simulink model "TractiveSystemCooling"  (R2023b)
settings: Solver=FixedStepAuto  StartTime=0.0  StopTime=runtime  FixedStep=.02  RelTol=1e-3
model workspace: external: MATLAB File Data/Settings.m (data not in the file)
undefined symbols (not defined in the file or in its folder): Cell, runtime, TSAC
libraries: fl_lib x5, nesl_utility x5, batteryecm_lib x1, dspstat3 x1
settings Model: Creator=13359

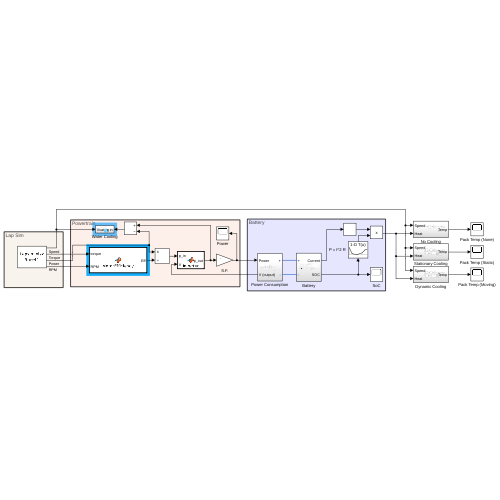
[thumbnail: Simulink's stored preview of the top-level diagram]
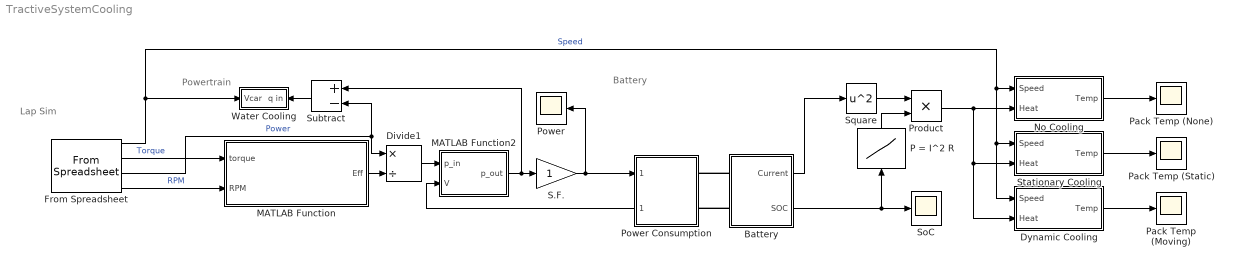
== system TractiveSystemCooling ==
  note: Powertrain
  note: Battery
  note: Lap Sim
  Battery : Subsystem
  Divide1 : Product  Inputs=*/
  Dynamic Cooling : Subsystem
  From Spreadsheet : FromSpreadsheet  FileName=Lapsim.xlsx  Range=E1:E5414, W1:Y5414  TreatFirstColumnAs=Data  SampleTime=0.02
  MATLAB Function : MATLAB Function  TreatAsAtomicUnit=on
  MATLAB Function2 : MATLAB Function  TreatAsAtomicUnit=on
  No Cooling : Subsystem
  P = I^2 R : Lookup_n-D  NumberOfTableDimensions=1  BreakpointsForDimension1=Cell.SOC  Table=zeros(1,length(Cell.SOC)) + (Cell.Resistance*Cell.series/Cell.parallel)  InternalRulePriority=Speed  RndMeth=Simplest
  Pack Temp (Moving) : Scope
  Pack Temp (None) : Scope
  Pack Temp (Static) : Scope
  Power : Scope
  Power Consumption : Subsystem
      settings: PortSchema="{\"entries\":[{\"content\":{\"sides\":[{\"content\":{\"connectorIds\":[\"In1\",\"Out1\"]},\"type\":\"ConnectorPlacement.EquallySpacedRectSide\",\"uuid\":\"bce31be9-9828-45d3-a0ec-acfed125f971\"},{\"content\":{\"connectorIds\":[\"RConn1\",\"RConn2\"],\"side\":\"RIGHT\"},\"type\":\"ConnectorPlacement.EquallySpacedRectSide\",\"uuid\":\"688da906-5253-49d4-8895-2a1ab7d3d08f\"},{\"content\":{\"side\":\"TOP\"},\"type\":\"ConnectorPlacement.EquallySpacedRectSide\",\"uuid\":\"26fec6ea-0e9b-46d7-ab73-190f763a0feb\"}]},\"type\":\"ConnectorPlacement.EquallySpacedConnector\",\"uuid\":\"dca3bc88-c6e8-4b99-b46a-70a0164d4b50\"}],\"packageUris\":[\"http://schema.mathworks.com/mf0/Connector/R2020b\"],\"version\":\"1.0\"}"
  Product : Product
  S.F. : Gain
  SoC : Scope
  Square : Math  Operator=square
  Stationary Cooling : Subsystem
  Subtract : Sum  Inputs=+-
  Water Cooling : Subsystem
      settings: PortSchema="{\"entries\":[{\"content\":{\"sides\":[{\"content\":{\"connectorIds\":[\"In1\"]},\"type\":\"ConnectorPlacement.EquallySpacedRectSide\",\"uuid\":\"7b584cd1-b16c-47c3-a77c-0f72b30f83a9\"},{\"content\":{\"connectorIds\":[\"In2\"],\"side\":\"RIGHT\"},\"type\":\"ConnectorPlacement.EquallySpacedRectSide\",\"uuid\":\"743ce824-323e-45dd-9a42-fd02d44e7a7c\"},{\"content\":{\"side\":\"TOP\"},\"type\":\"ConnectorPlacement.EquallySpacedRectSide\",\"uuid\":\"adabee87-d3a0-4ce2-a1ff-e6a273d4f474\"}]},\"type\":\"ConnectorPlacement.EquallySpacedConnector\",\"uuid\":\"782a8077-db8b-432e-a7e4-fc43f04762f2\"}],\"packageUris\":[\"http://schema.mathworks.com/mf0/Connector/R2020b\"],\"version\":\"1.0\"}"
  wires:
  MATLAB Function/1(Eff) -> Divide1/2
  From Spreadsheet/3 -> Divide1/1, Subtract/2  "Power"
  From Spreadsheet/2 -> MATLAB Function/1(torque)  "Torque"
  Square/1 -> Product/1
  From Spreadsheet/4 -> MATLAB Function/2(RPM)  "RPM"
  Product/1 -> Stationary Cooling/2(Heat), Dynamic Cooling/2(Heat), No Cooling/2(Heat)
  S.F./1 -> Power/1, Power Consumption/1(Power)
  From Spreadsheet/1 -> Dynamic Cooling/1(Speed), Stationary Cooling/1(Speed), No Cooling/1(Speed), Water Cooling/2(Vcar)  "Speed"
  Subtract/1 -> Water Cooling/1(q in)
  Divide1/1 -> MATLAB Function2/1(p_in)
  MATLAB Function2/1(p_out) -> S.F./1, Subtract/1
  Dynamic Cooling/1(Temp) -> Pack Temp (Moving)/1
  Stationary Cooling/1(Temp) -> Pack Temp (Static)/1
  No Cooling/1(Temp) -> Pack Temp (None)/1
  Battery/2(SOC) -> P = I^2 R/1, SoC/1
  Power Consumption/1(V (output)) -> MATLAB Function2/2(V)
  P = I^2 R/1 -> Product/2
  Battery/1(Current) -> Square/1
  connections:
  Battery/LConn2 -- Power Consumption/RConn2
  Battery/LConn1 -- Power Consumption/RConn1

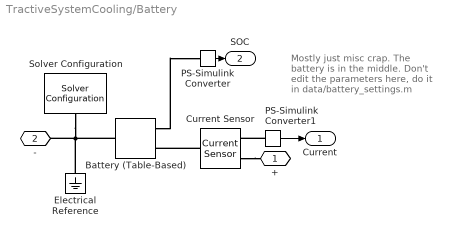
== system TractiveSystemCooling/Battery ==
  note: Mostly just misc crap.
      | The battery is in the
      | middle. Don't edit the
      | parameters here, do it
      | in data/battery_settings.m
  Battery (Table-Based) : batteryecm_lib/Battery (Table-Based)  SOC_vec=Cell.SOC  T_dependence=simscape.enum.tablebattery.temperature_dependence.no  prm_dir=simscape.enum.tablebattery.prm_dir.noCurrentDirectionality  T_vec=[278, 293, 313] K  V0_mat=[3.49, 3.5, 3.51; 3.55, 3.57, 3.56; 3.62, 3.63, 3.64; 3.71, 3.71, 3.72; 3.91, 3.93, 3.94; 4.07, 4.08, 4.08; 4.19, 4.19, 4.19] V  V0_vec=zeros(1,length(Cell.SOC)) + (Cell.V * Cell.series) V  V_range=[0, inf] V  R0_mat=[.0117, .0085, .009; .011, .0085, .009; .0114, .0087, .0092; .0107, .0082, .0088; .0107, .0083, .0091; .0113, .0085, .0089; .0116, .0085, .0089] Ohm  R0_vec=zeros(1,length(Cell.SOC)) + (Cell.Resistance*Cell.series/Cell.parallel) Ohm  R0_dis_mat=[.0117, .0085, .009; .011, .0085, .009; .0114, .0087, .0092; .0107, .0082, .0088; .0107, .0083, .0091; .0113, .0085, .0089; .0116, .0085, .0089] Ohm  R0_dis_vec=[.0085, .0085, .0087, .0082, .0083, .0085, .0085] Ohm  R0_ch_mat=[.0117, .0085, .009; .011, .0085, .009; .0114, .0087, .0092; .0107, .0082, .0088; .0107, .0083, .0091; .0113, .0085, .0089; .0116, .0085, .0089] Ohm  R0_ch_vec=[.0085, .0085, .0087, .0082, .0083, .0085, .0085] Ohm  AH=Cell.Capacity * Cell.parallel A*hr  prm_leak=simscape.enum.tablebattery.prm_leak.disabled  Rleak_vec=[8000, 7000, 6000] Ohm  Rleak=7e3 Ohm  extrapolation_option=simscape.enum.extrapolation.linear  SOC_port=simscape.enum.tablebattery.enable.yes  prm_dyn=simscape.enum.tablebattery.prm_dyn.off  R1_mat=[.0109, .0029, .0013; .0069, .0024, .0012; .0047, .0026, .0013; .0034, .0016, .001; .0033, .0023, .0014; .0033, .0018, .0011; .0028, .0017, .0011] Ohm  R1_vec=[.0029, .0024, .0026, .0016, .0023, .0018, .0017] Ohm  tau1_mat=[20, 36, 39; 31, 45, 39; 109, 105, 61; 36, 29, 26; 59, 77, 67; 40, 33, 29; 25, 39, 33] s  tau1_vec=[36, 45, 105, 29, 77, 33, 39] s  R2_mat=[.0109, .0029, .0013; .0069, .0024, .0012; .0047, .0026, .0013; .0034, .0016, .001; .0033, .0023, .0014; .0033, .0018, .0011; .0028, .0017, .0011] Ohm  R2_vec=[.0029, .0024, .0026, .0016, .0023, .0018, .0017] Ohm  tau2_mat=[20, 36, 39; 31, 45, 39; 109, 105, 61; 36, 29, 26; 59, 77, 67; 40, 33, 29; 25, 39, 33] s  tau2_vec=[36, 45, 105, 29, 77, 33, 39] s  R3_mat=[.0109, .0029, .0013; .0069, .0024, .0012; .0047, .0026, .0013; .0034, .0016, .001; .0033, .0023, .0014; .0033, .0018, .0011; .0028, .0017, .0011] Ohm  R3_vec=[.0029, .0024, .0026, .0016, .0023, .0018, .0017] Ohm  tau3_mat=[20, 36, 39; 31, 45, 39; 109, 105, 61; 36, 29, 26; 59, 77, 67; 40, 33, 29; 25, 39, 33] s  tau3_vec=[36, 45, 105, 29, 77, 33, 39] s  R4_mat=[.0109, .0029, .0013; .0069, .0024, .0012; .0047, .0026, .0013; .0034, .0016, .001; .0033, .0023, .0014; .0033, .0018, .0011; .0028, .0017, .0011] Ohm  R4_vec=[.0029, .0024, .0026, .0016, .0023, .0018, .0017] Ohm  tau4_mat=[20, 36, 39; 31, 45, 39; 109, 105, 61; 36, 29, 26; 59, 77, 67; 40, 33, 29; 25, 39, 33] s  tau4_vec=[36, 45, 105, 29, 77, 33, 39] s  R5_mat=[.0109, .0029, .0013; .0069, .0024, .0012; .0047, .0026, .0013; .0034, .0016, .001; .0033, .0023, .0014; .0033, .0018, .0011; .0028, .0017, .0011] Ohm  R5_vec=[.0029, .0024, .0026, .0016, .0023, .0018, .0017] Ohm  tau5_mat=[20, 36, 39; 31, 45, 39; 109, 105, 61; 36, 29, 26; 59, 77, 67; 40, 33, 29; 25, 39, 33] s  tau5_vec=[36, 45, 105, 29, 77, 33, 39] s  prm_fade=simscape.enum.tablebattery.prm_fade.disabled  N0=100  dV0=0  dR0=0  dAH=0  dRleak=0  dR1=0  dR2=0  dR3=0  dR4=0  dR5=0  N0vec=[0, 100, 200, 300]  Tfadevec=[298.15, 323.15] K  dV0vec=[0, 0, 0, 0]  dR0vec=[0, 0, 0, 0]  dAHvec=[0, 0, 0, 0]  dRleakvec=[0, 0, 0, 0]  dR1vec=[0, 0, 0, 0]  dR2vec=[0, 0, 0, 0]  dR3vec=[0, 0, 0, 0]  dR4vec=[0, 0, 0, 0]  dR5vec=[0, 0, 0, 0]  dV0mat=[0, 0; 0, 0; 0, 0; 0, 0]  dR0mat=[0, 0; 0, 0; 0, 0; 0, 0]  dAHmat=[0, 0; 0, 0; 0, 0; 0, 0]  dRleakmat=[0, 0; 0, 0; 0, 0; 0, 0]  dR1mat=[0, 0; 0, 0; 0, 0; 0, 0]  dR2mat=[0, 0; 0, 0; 0, 0; 0, 0]  dR3mat=[0, 0; 0, 0; 0, 0; 0, 0]  dR4mat=[0, 0; 0, 0; 0, 0; 0, 0]  dR5mat=[0, 0; 0, 0; 0, 0; 0, 0]  prm_age_modeling=simscape.enum.tablebattery.prm_age_modeling.equation  storage_dt_age_vec=[0] d  storage_T_age_vec=[273] K  prm_age_OCV=simscape.enum.tablebattery.prm_age_OCV.OCV  OCV_age=0.9  SOC_age=0.6  prm_age_resistance=simscape.enum.tablebattery.prm_age.disabled  OCV_scaling_age_resistance=2.2134e6  OCV_offset_age_resistance=1.632e6  temp_exp_age_resistance=0.515833569 V  t_exp_age_resistance=0.75  T_age_vec_resistance=[273.15, 298.15, 323.15] K  dt_age_vec_resistance=[0, 90, 180, 270] d  dR0_age_vec=[0, 0, 0]  t_meas_dR0_age=100 d  dR0_age_mat=[0, 0, 0; 0, 0, 0; 0, 0, 0; 0, 0, 0]  prm_age_capacity=simscape.enum.tablebattery.prm_age.disabled  OCV_scaling_age_capacity=1.5097e07  OCV_offset_age_capacity=8.3625e06  temp_exp_age_capacity=0.6011 V  t_exp_age_capacity=0.75  T_age_vec_capacity=[273.15, 298.15, 323.15] K  dt_age_vec_capacity=[0, 90, 180, 270] d  dAH_age_vec=[0, 0, 0]  t_meas_dAH_age=100 d  dAH_age_mat=[0, 0, 0; 0, 0, 0; 0, 0, 0; 0, 0, 0]  thermal_port=simscape.enum.thermaleffects.omit  temperature=298.15 K  thermal_mass=100 J/K  i_specify=off  i_priority=None  i=0 A  i_nominal_specify=off  i_nominal_unit=A  i_nominal_value=1  v_specify=off  v_priority=None  v=0 V  v_nominal_specify=off  v_nominal_unit=V  v_nominal_value=1  stateOfCharge_specify=off  stateOfCharge_priority=High  stateOfCharge=1  stateOfCharge_nominal_specify=off  stateOfCharge_nominal_unit=1  stateOfCharge_nominal_value=1  num_cycles_specify=off  num_cycles_priority=High  num_cycles=0  num_cycles_nominal_specify=off  num_cycles_nominal_unit=1  num_cycles_nominal_value=1  cell_temperature_specify=off  cell_temperature_priority=High  cell_temperature=298.15 K  cell_temperature_nominal_specify=off  cell_temperature_nominal_unit=K  cell_temperature_nominal_value=1
      settings: InternalSimscapePortConfiguration="{\"Bottom\":[],\"Left\":[{\"id\":\"p\",\"label\":\"+\",\"type\":\"foundation.electrical.electrical\"},{\"id\":\"soc\",\"label\":\"SOC\",\"type\":\"output\"}],\"Right\":[{\"id\":\"n\",\"label\":\"-\",\"type\":\"foundation.electrical.electrical\"}],\"Top\":[]}"
      settings: LibrarySourceBlock=|
      | batt_lib/Cells/Battery
      | (Table-Based)
  Current Sensor : fl_lib/Electrical/Electrical Sensors/Current Sensor
  Electrical Reference : fl_lib/Electrical/Electrical Elements/Electrical Reference
  PS-Simulink Converter : nesl_utility/PS-Simulink Converter  PhysicalDomain=network_engine_domain  SubClassName=ps_output  LeftPortType=input  RightPortType=output  PseudoPeriodic=off  Frequencies=[]  VectorFormat=inherit  Unit=inherit  AffineConversion=off
  PS-Simulink Converter1 : nesl_utility/PS-Simulink Converter  PhysicalDomain=network_engine_domain  SubClassName=ps_output  LeftPortType=input  RightPortType=output  PseudoPeriodic=off  Frequencies=[]  VectorFormat=inherit  Unit=inherit  AffineConversion=off
  Solver Configuration : nesl_utility/Solver Configuration  PhysicalDomain=network_engine_domain  SubClassName=solver  LeftPortType=input  RightPortType=generic  Tones=[]  Harmonics=[]  SimulateNoise=off  Profile=off  UseLocalSampling=off  EnableSwitchedLinearOptims=on  FrequencyDomain=off  UseCCode=off  RelTol=0.001  AbsTol=0.001  MinStep=1e-09  ToWorkspace=off  RevertToSquareIcSolve=off  NumHomotopyIterations=100  PhasorMode=off  PhasorModeNumHarmonics=1  ConsistencySolver=NEWTON_XTOL_AFTER_FTOL  IndexReductionMethod=DerivativeReplacement  DoDC=off  ResidualTolerance=1e-09  ConsistencyTolSource=GLOBAL  ConsistencyAbsTol=0.001  ConsistencyRelTol=0.001  ConsistencyTolFactor=0.001  UseLocalSolver=on  LocalSolverChoice=NE_BACKWARD_EULER_ADVANCER  ResolveIndetEquations=on  FunctionEvalNumThread=1  LocalSolverSampleTime=0.02  DoFixedCost=on  MaxNonlinIter=3  MaxModeIter=2  ComputeImpulses=off  ImpulseIterations=2  LinearAlgebra=auto  LinearAlgebraNumThread=0  EquationFormulation=NE_TIME_EF  DelaysMemoryBudget=1024  AutomaticFiltering=on  FilteringTimeConstant=0.001  PartitionStorageMethod=AS_NEEDED  PartitionMemoryBudget=1024  PartitionMethod=ROBUST  MultibodyUseLocalSolver=off  MultibodyLocalSolverChoice=ODE1  MultibodyLocalSolverSampleTime=0.001
  + : PMIOPort  Side=Left
  - : PMIOPort  Port=2  Side=Left
  Current : Outport
  SOC : Outport  Port=2
  wires:
  PS-Simulink Converter/1 -> SOC/1
  PS-Simulink Converter1/1 -> Current/1
  connections:
  Electrical Reference/LConn1 -- -/RConn1 -- Solver Configuration/RConn1 -- Battery (Table-Based)/RConn1
  Current Sensor/LConn1 -- Battery (Table-Based)/LConn1
  PS-Simulink Converter1/LConn1 -- Current Sensor/RConn1
  Current Sensor/RConn2 -- +/RConn1
  Battery (Table-Based)/LConn2 -- PS-Simulink Converter/LConn1

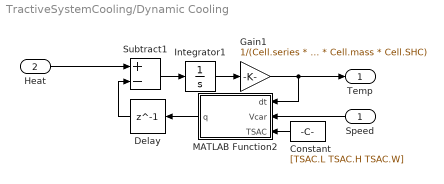
== system TractiveSystemCooling/Dynamic Cooling ==
  Speed : Inport
  Heat : Inport  Port=2
  Constant : Constant  Value=[TSAC.L TSAC.H TSAC.W]
  Delay : Delay  DelayLength=1
  Gain1 : Gain  Gain=1/(Cell.series * Cell.parallel * Cell.mass * Cell.SHC)
  Integrator1 : Integrator
  MATLAB Function2 : MATLAB Function  TreatAsAtomicUnit=on
  Subtract1 : Sum  Inputs=+-
  Temp : Outport
  wires:
  MATLAB Function2/1(q) -> Delay/1
  Delay/1 -> Subtract1/2
  Gain1/1 -> MATLAB Function2/1(dt), Temp/1
  Heat/1 -> Subtract1/1
  Subtract1/1 -> Integrator1/1
  Integrator1/1 -> Gain1/1
  Speed/1 -> MATLAB Function2/2(Vcar)
  Constant/1 -> MATLAB Function2/3(TSAC)

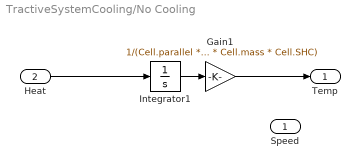
== system TractiveSystemCooling/No Cooling ==
  Speed : Inport
  Heat : Inport  Port=2
  Gain1 : Gain  Gain=1/(Cell.parallel * Cell.series * Cell.mass * Cell.SHC)
  Integrator1 : Integrator
  Temp : Outport
  wires:
  Gain1/1 -> Temp/1
  Heat/1 -> Integrator1/1
  Integrator1/1 -> Gain1/1

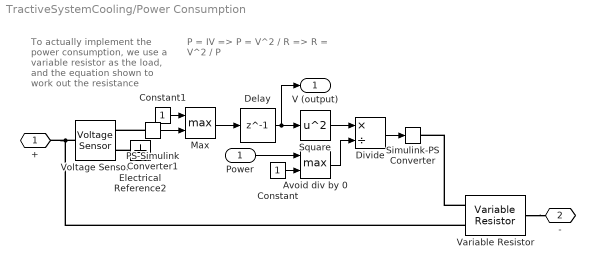
== system TractiveSystemCooling/Power Consumption ==
  note: To actually implement the
      | power consumption, we
      | use a variable resistor as
      | the load, and the equation
      | shown to work out the
      | resistance
  note: P = IV
      | => P = V^2 / R
      | => R = V^2 / P
  Power : Inport
  Avoid div by 0 : MinMax  Function=max  Inputs=2
  Constant : Constant
  Constant1 : Constant
  Delay : Delay  DelayLength=1  InitialCondition=445.2
  Divide : Product  Inputs=*/
  Electrical Reference2 : fl_lib/Electrical/Electrical Elements/Electrical Reference
  Max : MinMax  Function=max  Inputs=2
  PS-Simulink Converter1 : nesl_utility/PS-Simulink Converter  PhysicalDomain=network_engine_domain  SubClassName=ps_output  LeftPortType=input  RightPortType=output  PseudoPeriodic=off  Frequencies=[]  VectorFormat=inherit  Unit=inherit  AffineConversion=off
  Simulink-PS Converter : nesl_utility/Simulink-PS Converter  PhysicalDomain=network_engine_domain  SubClassName=ps_input  LeftPortType=input  RightPortType=output  PseudoPeriodic=off  Frequencies=[]  NoiseDistribution=none  NoiseParameters=[]  Unit=1  AffineConversion=off  FilteringAndDerivatives=provide  SimscapeFilterOrder=1  InputFilterTimeConstant=0.001  UdotUserProvided=0
  Square : Math  Operator=square
  Variable Resistor : fl_lib/Electrical/Electrical Elements/Variable Resistor  Rmin=0 Ohm  thermalEnable=false  thermal_mass=1 J/K  i_specify=off  i_priority=None  i=0 A  i_nominal_specify=off  i_nominal_unit=A  i_nominal_value=1  v_specify=off  v_priority=None  v=0 V  v_nominal_specify=off  v_nominal_unit=V  v_nominal_value=1  T_specify=off  T_priority=None  T=300 K  T_nominal_specify=off  T_nominal_unit=K  T_nominal_value=1
  Voltage Sensor : fl_lib/Electrical/Electrical Sensors/Voltage Sensor
  + : PMIOPort  Side=Right
  - : PMIOPort  Port=2  Side=Right
  V (output) : Outport
  wires:
  Square/1 -> Divide/1
  Delay/1 -> V (output)/1, Square/1
  Divide/1 -> Simulink-PS Converter/1
  Constant/1 -> Avoid div by 0/2
  Avoid div by 0/1 -> Divide/2
  Power/1 -> Avoid div by 0/1
  Max/1 -> Delay/1
  Constant1/1 -> Max/1
  PS-Simulink Converter1/1 -> Max/2
  connections:
  Electrical Reference2/LConn1 -- Voltage Sensor/RConn2
  PS-Simulink Converter1/LConn1 -- Voltage Sensor/RConn1
  Voltage Sensor/LConn1 -- Variable Resistor/LConn2 -- +/RConn1
  Variable Resistor/LConn1 -- Simulink-PS Converter/RConn1
  Variable Resistor/RConn1 -- -/RConn1

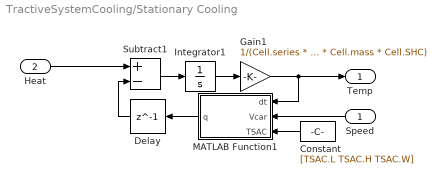
== system TractiveSystemCooling/Stationary Cooling ==
  Speed : Inport
  Heat : Inport  Port=2
  Constant : Constant  Value=[TSAC.L TSAC.H TSAC.W]
  Delay : Delay  DelayLength=1
  Gain1 : Gain  Gain=1/(Cell.series * Cell.parallel * Cell.mass * Cell.SHC)
  Integrator1 : Integrator
  MATLAB Function1 : MATLAB Function  TreatAsAtomicUnit=on
  Subtract1 : Sum  Inputs=+-
  Temp : Outport
  wires:
  MATLAB Function1/1(q) -> Delay/1
  Delay/1 -> Subtract1/2
  Gain1/1 -> Temp/1, MATLAB Function1/1(dt)
  Heat/1 -> Subtract1/1
  Subtract1/1 -> Integrator1/1
  Integrator1/1 -> Gain1/1
  Speed/1 -> MATLAB Function1/2(Vcar)
  Constant/1 -> MATLAB Function1/3(TSAC)

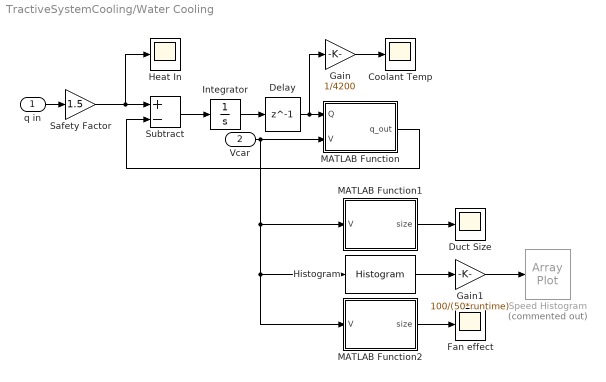
== system TractiveSystemCooling/Water Cooling ==
  q in : Inport
  Vcar : Inport  Port=2
  Coolant Temp : Scope
  Delay : Delay  DelayLength=1  InitialCondition=20*4200
  Duct Size : Scope
  Fan effect : Scope
  Gain : Gain  Gain=1/4200
  Gain1 : Gain  Gain=100/(50*runtime)
  Heat In : Scope
  Histogram : dspstat3/Histogram  umin=0  umax=40  nbins=41  operateOver=Each column  Dimension=1  normalized=off  run=on  reset=on  trigtype=None  colComp=on  roundingMode=Floor  overflowMode=off
  Integrator : Integrator  InitialCondition=4200*20
  MATLAB Function : MATLAB Function  TreatAsAtomicUnit=on
  MATLAB Function1 : MATLAB Function  TreatAsAtomicUnit=on
  MATLAB Function2 : MATLAB Function  TreatAsAtomicUnit=on
  Safety Factor : Gain  Gain=1.5
  Speed Histogram : ArrayPlot  Commented=on  WindowPosition=[196.000000,35.000000,800.000000,500.000000,]  ScopeFrameLocation=window  YLimits=[-0.125 1.125]
  Subtract : Sum  Inputs=+-
  wires:
  Gain/1 -> Coolant Temp/1
  Subtract/1 -> Integrator/1
  Integrator/1 -> Delay/1
  Delay/1 -> Gain/1, MATLAB Function/1(Q)
  MATLAB Function/1(q_out) -> Subtract/2
  q in/1 -> Safety Factor/1
  Safety Factor/1 -> Heat In/1, Subtract/1
  Vcar/1 -> MATLAB Function2/1(V), Histogram/1, MATLAB Function1/1(V), MATLAB Function/2(V)
  MATLAB Function1/1(size) -> Duct Size/1
  Histogram/1 -> Gain1/1
  Gain1/1 -> Speed Histogram/1
  MATLAB Function2/1(size) -> Fan effect/1

== matlab function TractiveSystemCooling/Water Cooling/MATLAB Function1 ==
  data: size output; V input
function size = fcn(V)
state = Radiator_settings;
state.V_car = V;
size = Airflow(state)/(state.radiator.H*state.radiator.L*V);

== matlab function TractiveSystemCooling/MATLAB Function ==
  data: torque input; RPM input; Eff output
function Eff = MotorEfficiency(torque, RPM)
    % Emrax 208. If you ever change motor, use PyOpenCV and numpy/MATLAB
    % polyfit to make something like this for the new one, using the
    % efficiency contour from the datasheet (if there is one). This should 
    % return a value in [0,1] 
    p00 =       85.36;
    p10 =   -0.004406;
    p01 =     -0.2588;
    p20 =   3.797e-06;
    p11 =   0.0004744;
    p02 =     0.01083;
    p30 =  -1.928e-09;
    p21 =  -1.306e-07;
    p12 =  -4.173e-06;
    p03 =   -0.000191;
    p40 =   4.758e-13;
    p31 =   1.263e-11;
    p22 =   6.055e-10;
    p13 =   2.415e-08;
    p04 =   1.333e-06;
    p50 =  -4.838e-17;
    p41 =   1.036e-15;
    p32 =  -1.164e-13;
    p23 =   1.444e-12;
    p14 =  -9.625e-11;
    p05 =   -3.18e-09;

    Eff = p00 + p10*RPM + p01*torque + p20*RPM^2 + p11*RPM*torque + p02*torque^2 + p30*RPM^3 + p21*RPM^2*torque ...
    + p12*RPM*torque^2 + p03*torque^3 + p40*RPM^4 + p31*RPM^3*torque + p22*RPM^2*torque^2 ...
    + p13*RPM*torque^3 + p04*torque^4 + p50*RPM^5 + p41*RPM^4*torque + p32*RPM^3*torque^2 ...
    + p23*RPM^2*torque^3 + p14*RPM*torque^4 + p05*torque^5;
    Eff = Eff / 100;
    Eff = max(Eff, 0.8);
end

== matlab function TractiveSystemCooling/Water Cooling/MATLAB Function ==
  data: Q input; q_out output; V input
function q_out = fcn(Q, V)

q_out = Rate(Q/4200, V);

== matlab function TractiveSystemCooling/MATLAB Function2 ==
  data: p_in input; p_out output; V input
function p_out = Inverter(p_in, V)

% Inverter inefficiency is tabulated vs V and I, so we implement that here

p_out = p_in + interp2([50 100 150 200 250 300 350], [200 400 600 800], ...
    [129 261 402 552 717 894 1083; ...
     201 384 579 783 999 1233 1479; ...
     270 513 759 1020 1290 1584 1899; ...
     342 642 945 1260 1596 1956 2343], ...
     p_in/V, V, 'spline');

== matlab function TractiveSystemCooling/Dynamic Cooling/MATLAB Function2 ==
  data: dt input; Vcar input; q output; TSAC input
function q = Cooling(dt, Vcar, TSAC)

function G = Gr(dt, L) % Grashof Number
    G = (9.81*(1/(293.15+dt))*dt*L^3)/(15.69e-6)^2;
end
Pr = 0.71; % Prandtl Number
k = .026;  % Conductivity of air

% Basic TSAC Dimensions
L = TSAC(1);
H = TSAC(2);
W = TSAC(3);

% Area of each face of the TSAC
A_t = L*W;
A_s3 = 2*W*H;
A_s6 = 2*L*H;
A_b = L*W;

% Hydraulic Radii
r_t  = A_t  / (2*(L+W));
r_s3 = A_s3 / (2*(W+H));
r_s6 = A_s6 / (2*(L+H));
r_b  = A_b  / (2*(L+W));

%Rayleigh Numbers
Ra_t = Gr(dt, r_t)*Pr;
Ra_s = Gr(dt, H)*Pr;
Ra_b = Gr(dt, r_b)*Pr;

% Conductive heat transfer coeffs
h_t =  .54*Ra_t^(1/4) * k/r_t;
h_s3 = .59*Ra_s^(1/4) * k/r_s3;
h_s6 = .59*Ra_s^(1/4) * k/r_s6;
h_b =  .27*Ra_b^(1/4) * k/r_b;

hA = h_t*A_t + h_s3*A_s3 + h_s6*A_s6 + h_b*A_b; % Natural Convection


%% With Vcar
% Characteristic Lengths
L_b = W;
L_s = H;

% Reynolds Numbers
Re_b = 1.2 * Vcar * L_b / 1.8e-5;
Re_s = 1.2 * Vcar * L_s / 1.8e-5;

% Nusselt Numbers
Nu_b = .023 * Re_b^0.8 * Pr^.4;
Nu_s = .023 * Re_s^0.8 * Pr^.4;

% Heat coeffs
h_b = Nu_b * k / L_b;
h_s = Nu_s * k / L_s;
hA = h_b*A_b + h_s*A_s6 + h_s3*A_s3 + h_t*A_t;

q = hA*dt;
q = q + (5.669e-8)*((293.15+dt)^4-293.15^4)*(A_t + A_s3 +A_s6 + A_b); % Radiation
end

== matlab function TractiveSystemCooling/Stationary Cooling/MATLAB Function1 ==
  data: dt input; Vcar input; q output; TSAC input
function q = Cooling(dt, Vcar, TSAC)

function G = Gr(dt, L) % Grashof Number
    G = (9.81*(1/(293.15+dt))*dt*L^3)/(15.69e-6)^2;
end
Pr = 0.71; % Prandtl Number
k = .026;  % Conductivity of air

% Basic TSAC Dimensions
L = TSAC(1);
H = TSAC(2);
W = TSAC(3);

% Area of each face of the TSAC
A_t = L*W;
A_s3 = 2*W*H;
A_s6 = 2*L*H;
A_b = L*W;

% Hydraulic Radii
r_t  = A_t  / (2*(L+W));
r_s3 = A_s3 / (2*(W+H));
r_s6 = A_s6 / (2*(L+H));
r_b  = A_b  / (2*(L+W));

%Rayleigh Numbers
Ra_t = Gr(dt, r_t)*Pr;
Ra_s = Gr(dt, H)*Pr;
Ra_b = Gr(dt, r_b)*Pr;

% Conductive heat transfer coeffs
h_t =  .54*Ra_t^(1/4) * k/r_t;
h_s3 = .59*Ra_s^(1/4) * k/r_s3;
h_s6 = .59*Ra_s^(1/4) * k/r_s6;
h_b =  .27*Ra_b^(1/4) * k/r_b;

hA = h_t*A_t + h_s3*A_s3 + h_s6*A_s6 + h_b*A_b; % Natural Convection

q = hA*dt;
q = q + (5.669e-8)*((293.15+dt)^4-293.15^4)*(A_t + A_s3 +A_s6 + A_b); % Radiation
end

== matlab function TractiveSystemCooling/Water Cooling/MATLAB Function2 ==
  data: size output; V input
function size = fcn(V)
state = Radiator_settings;
state.V_car = V;
size = Airflow(state)/(state.radiator.H*state.radiator.L*V);

size = size/.244 - 1;
